simulink model "project2_2015b"  (R2017b)
settings: Solver=ode15s  StartTime=0.0  StopTime=20  FixedStep=1  MaxStep=0.01  MinStep=1e-20  RelTol=1e-3  AbsTol=1e-3  EnableMultiTasking=on
values from neighbouring files (symbols this model uses):
  A_F = 2.33    [init.m]
  C_0 = 0.00475    [init.m]
  C_D = 0.26    [init.m]
  F_trac_max = T_mot_max/(G_fd*r_wheel)    (= 5295.82687518)    [init.m]
  full_throttle = [1000 1198 1502 1888 2502 3000 3500 4000 76 84 91 97 ... (40 elements, 8x5)]    [full_throttle.mat]
  g = 9.8    [init.m]
  G_fd = 0.2431    [init.m]    (also in kinetic_energy.m)
  M_veh = 1361 +100    (= 1461)    [init.m]    (also in kinetic_energy.m)
  mps_to_mph = 1/0.44704    (= 2.23693629205)    [init.m]
  N_r = 78    [init.m]    (also in kinetic_energy.m)
  N_s = 30    [init.m]    (also in kinetic_energy.m)
  optimum_bsfc = [1178 1172 1160 1166 1178 1166 1172 1184 1172 1184 1281 1688 ... (75 elements, 15x5)]    [optimum_bsfc.mat]
  P_gen_max = 30000    [init.m]
  P_mot_max = 50000    [init.m]
  r_wheel = 0.3107    [init.m]    (also in kinetic_energy.m)
  radps_to_rpm = 3600/377    (= 9.54907161804)    [init.m]
  rho = 1.225    [init.m]
  T_gen_max = 240    [init.m]
  T_mot_max = 400    [init.m]
  w_eng_max = 5000 * 2*pi/60    (= 523.598775598)    [init.m]
  w_eng_min = 1000 * 2*pi/60    (= 104.71975512)    [init.m]
  w_gen_max = 9000 * 2*pi/60    (= 942.477796077)    [init.m]
  w_gen_min = -10000 * 2*pi/60    (= -1047.1975512)    [init.m]
libraries: simulink x1
settings Model: Creator=wasynczu  LastModifiedBy=khan1
settings SolverCC: InitialStep=1e-20  SolverJacobianMethodControl=FullAnalytical  ZeroCrossAlgorithm=Adaptive  SolverResetMethod=Robust
settings DataIOCC: LimitDataPoints=on  SaveFormat=Array  SignalLoggingSaveFormat=ModelDataLogs
settings OptimizationCC: ExpressionDepthLimit=2147483647  LifeSpan=inf
settings DebuggingCC: WriteAfterReadMsg=EnableAllAsError  SolverPrmCheckMsg=warning  FcnCallInpInsideContextMsg=warning  AllowSymbolicDim=off  StateNameClashWarn=warning  SFUnexpectedBacktrackingDiag=warning  SFNoUnconditionalDefaultTransitionDiag=warning  SFExecutionAtInitializationDiag=none
settings HardwareCC: ProdBitPerPointer=32  ProdBitPerSizeT=32  ProdBitPerPtrDiffT=32  ProdLargestAtomicFloat=None  ProdIntDivRoundTo=Undefined  ProdEndianess=Unspecified  ProdWordSize=32  ProdHWDeviceType=32-bit Generic
settings ModelReferenceCC: PropagateSignalLabelsOutOfModel=off
settings CodeAppCC: StateflowObjectComments=on
settings GRTTargetCC: TargetLangStandard=C89/C90 (ANSI)  GeneratePreprocessorConditionals=Disable all  CombineOutputUpdateFcns=off  GRTInterface=on
settings ConfigComp: CovMetricSettings=dw  CovHtmlReporting=on  CovSaveCumulativeToWorkspaceVar=on  CovSaveSingleToWorkspaceVar=on  CovExternalEMLEnable=off  CovSFcnEnable=off

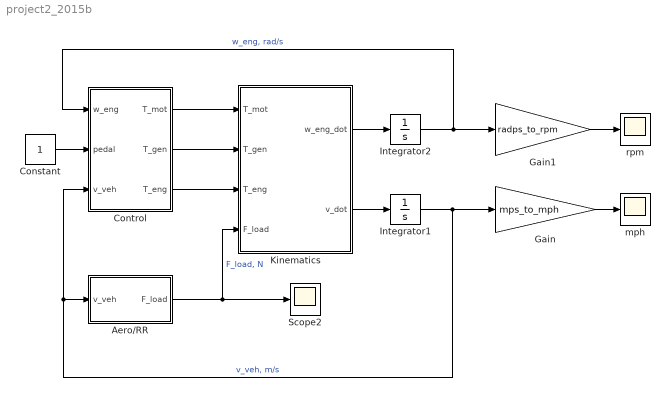
== system project2_2015b ==
  Aero/RR : Subsystem  mask{g=g, M_veh=M_veh, C_drag=C_D, A=A_F, C_rr=C_0, rho=rho}
      mask prompts: g "Earth acceleration, m/s^2"; M_veh "Vehicle mass, kg"; C_drag "Drag coefficient"; A "Frontal area, m^2"; C_rr "Rolling resistance coeeficient"; rho "Air density, kg/m^3"
  Constant : Constant
  Control : Subsystem
  Gain : Gain  Gain=mps_to_mph
  Gain1 : Gain  Gain=radps_to_rpm
  Integrator1 : Integrator
  Integrator2 : Integrator
  Kinematics : MATLAB Function  TreatAsAtomicUnit=on
  Scope2 : Scope
  mph : Scope
  rpm : Scope
  wires:
  Kinematics/2(v_dot) -> Integrator1/1
  Integrator1/1 -> Control/3(v_veh), Aero/RR/1(v_veh), Gain/1  "v_veh, m/s"
  Aero/RR/1(F_load) -> Kinematics/4(F_load), Scope2/1  "F_load, N"
  Control/1(T_mot) -> Kinematics/1(T_mot)
  Control/2(T_gen) -> Kinematics/2(T_gen)
  Kinematics/1(w_eng_dot) -> Integrator2/1
  Integrator2/1 -> Control/1(w_eng), Gain1/1  "w_eng, rad/s"
  Constant/1 -> Control/2(pedal)
  Gain/1 -> mph/1
  Control/3(T_eng) -> Kinematics/3(T_eng)
  Gain1/1 -> rpm/1

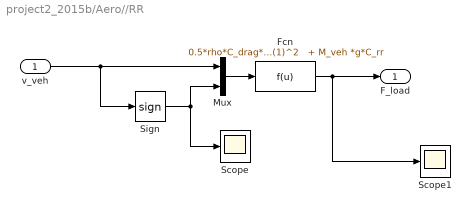
== system project2_2015b/Aero//RR ==
  v_veh : Inport
  Fcn : Fcn  Expr="0.5*rho*C_drag*A*u(1)^2   + M_veh *g*C_rr"
  Mux : Mux  Inputs=2
  Scope : Scope
  Scope1 : Scope
  Sign : Signum  ZeroCross=off
  F_load : Outport
  wires:
  Fcn/1 -> Scope1/1, F_load/1
  Mux/1 -> Fcn/1
  v_veh/1 -> Mux/1, Sign/1
  Sign/1 -> Mux/2, Scope/1

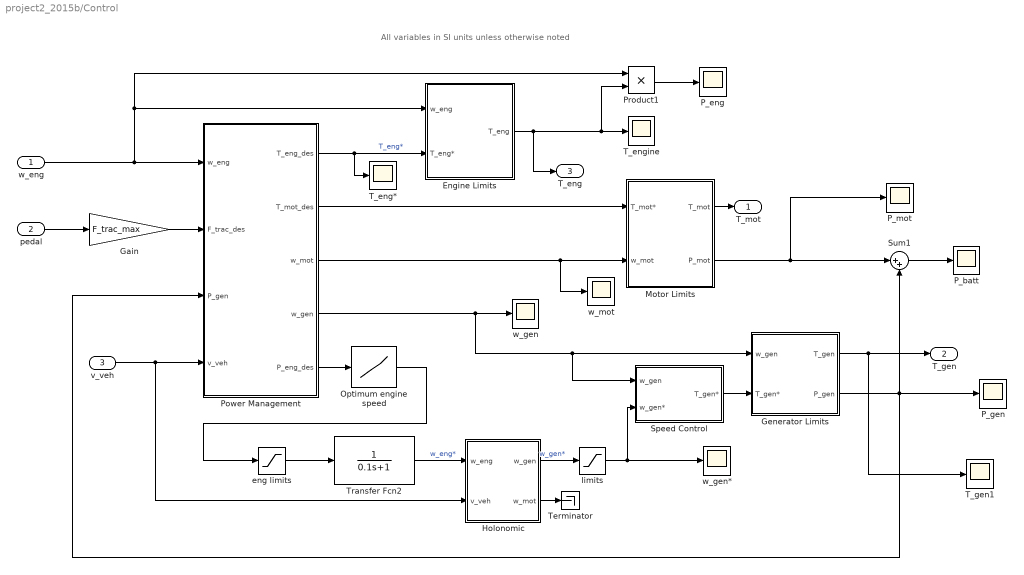
== system project2_2015b/Control ==
  note: All variables in SI units unless otherwise noted
  w_eng : Inport
  pedal : Inport  Port=2
  v_veh : Inport  Port=3
  Engine Limits : Subsystem
  Gain : Gain  Gain=F_trac_max
  Generator Limits : Subsystem
  Holonomic : Subsystem
  Motor Limits : Subsystem
  Optimum engine speed : Lookup_n-D  NumberOfTableDimensions=1  BreakpointsForDimension1=optimum_bsfc(:,5)  Table=optimum_bsfc(:,4)  InternalRulePriority=Speed  RndMeth=Simplest  InputSameDT=on
  P_batt : Scope
  P_eng : Scope
  P_gen : Scope
  P_mot : Scope
  Power Management : MATLAB Function  TreatAsAtomicUnit=on
  Product1 : Product
  Speed Control : Subsystem
  Sum1 : Sum  Inputs=|++
  T_eng* : Scope
  "T_engine " : Scope
  T_gen1 : Scope
  Terminator : Terminator
  Transfer Fcn2 : TransferFcn  Denominator=[0.1 1]
  eng limits : Saturate  UpperLimit=w_eng_max  LowerLimit=w_eng_min
  limits : Saturate  UpperLimit=w_gen_max  LowerLimit=w_gen_min
  w_gen : Scope
  w_gen* : Scope
  "w_mot " : Scope
  T_mot : Outport
  T_gen : Outport  Port=2
  T_eng : Outport  Port=3
  wires:
  pedal/1 -> Gain/1
  Power Management/4(w_gen) -> Speed Control/1(w_gen), Generator Limits/1(w_gen), w_gen/1
  Power Management/3(w_mot) -> "w_mot "/1, Motor Limits/2(w_mot)
  Motor Limits/1(T_mot) -> T_mot/1
  Speed Control/1(T_gen*) -> Generator Limits/2(T_gen*)
  Holonomic/1(w_gen) -> limits/1  "w_gen*"
  Gain/1 -> Power Management/2(F_trac_des)
  v_veh/1 -> Holonomic/2(v_veh), Power Management/4(v_veh)
  Power Management/1(T_eng_des) -> T_eng*/1, Engine Limits/2(T_eng*)  "T_eng*"
  Power Management/2(T_mot_des) -> Motor Limits/1(T_mot*)
  w_eng/1 -> Product1/1, Engine Limits/1(w_eng), Power Management/1(w_eng)
  Motor Limits/2(P_mot) -> Sum1/1, P_mot/1
  Sum1/1 -> P_batt/1
  Generator Limits/1(T_gen) -> T_gen1/1, T_gen/1
  Engine Limits/1(T_eng) -> "T_engine "/1, Product1/2, T_eng/1
  Generator Limits/2(P_gen) -> Power Management/3(P_gen), P_gen/1, Sum1/2
  Optimum engine speed/1 -> eng limits/1
  eng limits/1 -> Transfer Fcn2/1
  Product1/1 -> P_eng/1
  Holonomic/2(w_mot) -> Terminator/1
  Transfer Fcn2/1 -> Holonomic/1(w_eng)  "w_eng*"
  Power Management/5(P_eng_des) -> Optimum engine speed/1
  limits/1 -> Speed Control/2(w_gen*), w_gen*/1

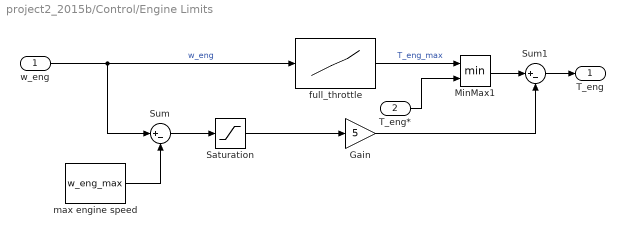
== system project2_2015b/Control/Engine Limits ==
  w_eng : Inport
  T_eng* : Inport  Port=2
  Gain : Gain  Gain=5
  MinMax1 : MinMax  Inputs=2
  Saturation : Saturate  UpperLimit=inf  LowerLimit=0
  Sum : Sum  Inputs=|+-
  Sum1 : Sum  Inputs=|+-
  full_throttle : Lookup_n-D  NumberOfTableDimensions=1  BreakpointsForDimension1=full_throttle(:,4)  Table=full_throttle(:,2)  InternalRulePriority=Speed  RndMeth=Simplest  InputSameDT=on
  max engine speed : Constant  Value=w_eng_max
  T_eng : Outport
  wires:
  w_eng/1 -> Sum/1, full_throttle/1  "w_eng"
  T_eng*/1 -> MinMax1/2
  full_throttle/1 -> MinMax1/1  "T_eng_max"
  max engine speed/1 -> Sum/2
  Sum/1 -> Saturation/1
  Sum1/1 -> T_eng/1
  MinMax1/1 -> Sum1/1
  Saturation/1 -> Gain/1
  Gain/1 -> Sum1/2

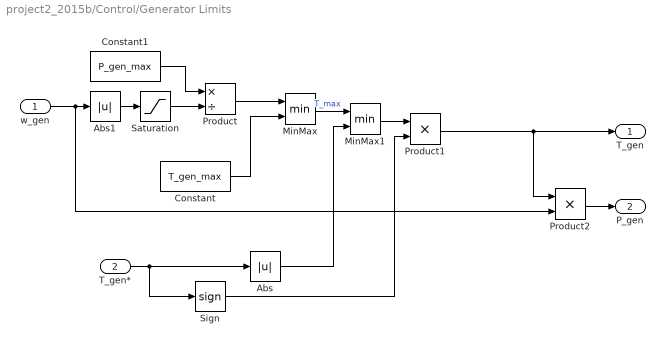
== system project2_2015b/Control/Generator Limits ==
  w_gen : Inport
  T_gen* : Inport  Port=2
  Abs : Abs
  Abs1 : Abs
  Constant : Constant  Value=T_gen_max  SampleTime=-1
  Constant1 : Constant  Value=P_gen_max
  MinMax : MinMax  Inputs=2
  MinMax1 : MinMax  Inputs=2
  Product : Product  Inputs=*/
  Product1 : Product
  Product2 : Product
  Saturation : Saturate  UpperLimit=inf  LowerLimit=0.01
  Sign : Signum
  T_gen : Outport
  P_gen : Outport  Port=2
  wires:
  Saturation/1 -> Product/2
  Product/1 -> MinMax/1
  Constant/1 -> MinMax/2
  Constant1/1 -> Product/1
  MinMax/1 -> MinMax1/1  "T_max"
  T_gen*/1 -> Sign/1, Abs/1
  Abs/1 -> MinMax1/2
  MinMax1/1 -> Product1/1
  Sign/1 -> Product1/2
  Abs1/1 -> Saturation/1
  Product1/1 -> Product2/1, T_gen/1
  Product2/1 -> P_gen/1
  w_gen/1 -> Product2/2, Abs1/1

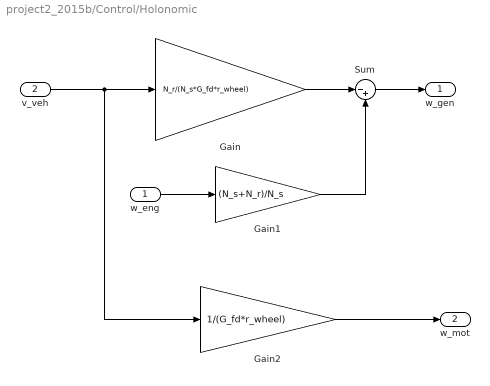
== system project2_2015b/Control/Holonomic ==
  w_eng : Inport
  v_veh : Inport  Port=2
  Gain : Gain  Gain=N_r/(N_s*G_fd*r_wheel)
  Gain1 : Gain  Gain=(N_s+N_r)/N_s
  Gain2 : Gain  Gain=1/(G_fd*r_wheel)
  Sum : Sum  Inputs=|-+
  w_gen : Outport
  w_mot : Outport  Port=2
  wires:
  Sum/1 -> w_gen/1
  v_veh/1 -> Gain2/1, Gain/1
  Gain/1 -> Sum/1
  w_eng/1 -> Gain1/1
  Gain1/1 -> Sum/2
  Gain2/1 -> w_mot/1

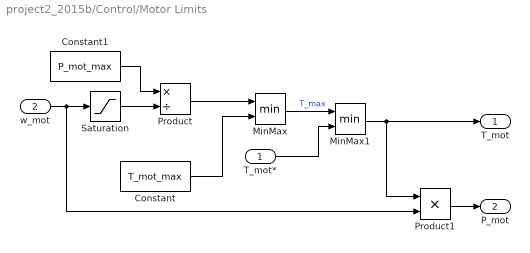
== system project2_2015b/Control/Motor Limits ==
  T_mot* : Inport
  w_mot : Inport  Port=2
  Constant : Constant  Value=T_mot_max
  Constant1 : Constant  Value=P_mot_max
  MinMax : MinMax  Inputs=2
  MinMax1 : MinMax  Inputs=2
  Product : Product  Inputs=*/
  Product1 : Product
  Saturation : Saturate  UpperLimit=inf  LowerLimit=0.01
  T_mot : Outport
  P_mot : Outport  Port=2
  wires:
  w_mot/1 -> Product1/2, Saturation/1
  Saturation/1 -> Product/2
  Product/1 -> MinMax/1
  Constant/1 -> MinMax/2
  Constant1/1 -> Product/1
  MinMax/1 -> MinMax1/1  "T_max"
  T_mot*/1 -> MinMax1/2
  Product1/1 -> P_mot/1
  MinMax1/1 -> T_mot/1, Product1/1

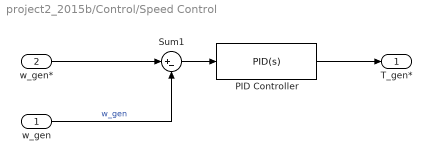
== system project2_2015b/Control/Speed Control ==
  w_gen : Inport
  w_gen* : Inport  Port=2
  PID Controller : simulink/Continuous/PID Controller  Controller=PID  TimeDomain=Continuous-time  SampleTime=-1  IntegratorMethod=Forward Euler  FilterMethod=Forward Euler  Form=Parallel  UseFilter=on  ControllerParametersSource=internal  P=100  I=1  D=0  N=100  InitialConditionSource=internal  InitialConditionForIntegrator=0  InitialConditionForFilter=0  ExternalReset=none  LimitOutput=off  UpperSaturationLimit=inf  LowerSaturationLimit=-inf  LinearizeAsGain=on  AntiWindupMode=none  Kb=1  TrackingMode=off  Kt=1  PParamMin=[]  PParamMax=[]  IParamMin=[]  IParamMax=[]  DParamMin=[]  DParamMax=[]  NParamMin=[]  NParamMax=[]  KbParamMin=[]  KbParamMax=[]  KtParamMin=[]  KtParamMax=[]  POutMin=[]  POutMax=[]  IOutMin=[]  IOutMax=[]  DOutMin=[]  DOutMax=[]  NOutMin=[]  NOutMax=[]  KbOutMin=[]  KbOutMax=[]  KtOutMin=[]  KtOutMax=[]  IntegratorOutMin=[]  IntegratorOutMax=[]  FilterOutMin=[]  FilterOutMax=[]  SumOutMin=[]  SumOutMax=[]  SumI1OutMin=[]  SumI1OutMax=[]  SumI2OutMin=[]  SumI2OutMax=[]  SumI3OutMin=[]  SumI3OutMax=[]  SumDOutMin=[]  SumDOutMax=[]  SaturationOutMin=[]  SaturationOutMax=[]  IntegratorContinuousStateAttributes=''  IntegratorStateMustResolveToSignalObject=off  IntegratorRTWStateStorageClass=Auto  FilterContinuousStateAttributes=''  FilterStateMustResolveToSignalObject=off  FilterRTWStateStorageClass=Auto  DifferentiatorICPrevScaledInput=0  DifferentiatorOutMin=[]  DifferentiatorOutMax=[]  InitialConditionSetting=State (most efficient)  FilterDiffOutCoefMin=[]  FilterDiffOutCoefMax=[]  SumDenOutMin=[]  SumDenOutMax=[]  SumNumOutMin=[]  SumNumOutMax=[]  ReciprocalOutMin=[]  ReciprocalOutMax=[]  DivideOutMin=[]  DivideOutMax=[]  TunerSelectOption=Transfer Function Based (PID Tuner App)
  Sum1 : Sum  Inputs=|+-
  T_gen* : Outport
  wires:
  Sum1/1 -> PID Controller/1
  PID Controller/1 -> T_gen*/1
  w_gen/1 -> Sum1/2  "w_gen"
  w_gen*/1 -> Sum1/1

== matlab function project2_2015b/Control/Power Management ==
  data: w_eng input; F_trac_des input; P_gen input; T_eng_des output; v_veh input; T_mot_des output; w_mot output; Param parameter; w_gen output; P_eng_des output
function [T_eng_des, T_mot_des, w_mot, w_gen, P_eng_des]  = fcn(w_eng, F_trac_des,  P_gen, v_veh, Param)
%#codegen

N_s = Param.N_s;            % number of sun teeth
N_r = Param.N_r;            % number of ring teeth
G_fd = Param.G_fd;
r_wheel = Param.r_wheel;
P_batt_max = Param.P_batt_max;
P_eng_max = Param.P_eng_max;
w_eng_min = Param.w_eng_min;

% Assume P_batt = P_batt_max for maximum acceleration

w_gen = w_eng*(N_r+N_s)/N_s - v_veh*N_r/(N_s*G_fd*r_wheel);
w_mot = v_veh/(G_fd*r_wheel);

P_trac_des = F_trac_des*v_veh;

if(P_trac_des < P_batt_max) % electric launch
    T_eng_des = 0;
    P_eng_des = 0;
    T_mot_des = F_trac_des * G_fd * r_wheel;
    P_mot_des = T_mot_des*w_mot;
    
    P_batt_des = P_mot_des + P_gen;

    if(P_batt_des > P_batt_max)
       P_mot_des = P_batt_max - P_gen;
       T_mot_des = P_mot_des/w_mot;
    end
 
   return
end

P_eng_des = P_trac_des - P_batt_max;
T_eng_des = P_eng_des/max([w_eng w_eng_min]);

if(P_eng_des > P_eng_max)
    P_eng_des = P_eng_max;
    T_eng_des = P_eng_des/max([w_eng w_eng_min]);
end

% calculate T_mot_des given P_batt and F_trac

A = [w_gen w_mot; -N_r/(N_s*G_fd*r_wheel) 1/(G_fd*r_wheel)];
b = [P_batt_max; F_trac_des];
x = A\b;
T_mot_des = x(2);

%check to see that P_batt will be less than P_batt_max

P_mot_des = T_mot_des * w_mot;
P_batt_des = P_mot_des + P_gen;

if(P_batt_des > P_batt_max)
   P_mot_des = P_batt_max - P_gen;
   T_mot_des = P_mot_des/w_mot;
end

return

== matlab function project2_2015b/Kinematics ==
  data: w_eng_dot output; T_mot input; T_gen input; T_eng input; F_load input; v_dot output; Param parameter
function [w_eng_dot, v_dot] = fcn(T_mot, T_gen, T_eng, F_load, Param)

N_s = Param.N_s; % number of sun teeth
N_r = Param.N_r; % number of ring teeth
G_fd = Param.G_fd; % gear ratio between motor and wheel speeds
r_wheel = Param.r_wheel; % wheel radius in m
Ainv = Param.Ainv; % inverse of state matrix A

% calculate generalized forces
Q_1 = (T_eng + T_gen*(N_s+N_r)/N_s);
Q_2 = (-F_load - T_gen*N_r/N_s/G_fd/r_wheel + T_mot/G_fd/r_wheel);

Q = [Q_1; Q_2];

y = Ainv * Q;

w_eng_dot = y(1);
v_dot = y(2);
